simulink model "Q0107tsmc_egtsmc_egftsmc_final_sensitivity"  (R2024b)
settings: Solver=ode4  StartTime=0.0  StopTime=12  FixedStep=0.01  RelTol=1e-3  EnableMultiTasking=on
model workspace (MAT data in the model file):
  A1 = 0.0190784648009
  A2 = 0.089786568484
  B1 = 2.58582251419
  B2 = 0.593361860386
  Count = 20
  I1 = 0.276
  I2 = 0.0235
  I3 = 0.0235
  L1 = 0.5
  L2 = 0.4
  Lp1d = 0.49
  Lp2d = 0.39
  Lp3d = 0.39
  Tmax = 0
  Tmin = -1567
  alpha1 = 1.4711
  alpha2 = 1.4464
  b10 = 33.49
  b11 = 1.435
  b12 = 3.205e-06
  b13 = -161.2
  b14 = 3.294
  b15 = -1.575e-05
  d10 = -0.78
  d11 = -76.79
  d20 = -0.4716
  d21 = 0.47
  dq = [1.72653408644e-22 0.000273900412394 0.000547772970539 0.000821597382973 0.00109535342539 0.0013690210252 0.00164258022129 0.0019160110909 0.00218929391546 0.0024624089498 0.00273533666065 0.00300805756768 ... (1200 elements, 400x3)]
  f10 = 0.0038
  f11 = 141.13
  f20 = 0.0012
  f21 = 150.24
  fai1d = 0.03998
  fai2d = 0.01996
  fai3d = 0.01996
  fce10 = 164.4
  fec11 = 0.003852
  fec12 = -0.9149
  g = 9.8
  ii = -1
  jj = 1
  k10 = 13640
  k11 = 0.05356
  k12 = -37.89
  kk = -1
  ks1 = 394.1176
  ks2 = 379.0476
  ll = 0
  m1 = 3.612
  m2 = 1.762
  nn = 0.1
  out = Simulink.SimulationOutput
  out.Data.e1a1 = [0 0.001 0.002 0.003 0.004 0.005 0.006 0.007 0.008 0.009 0.01 0.011 ... (100002 elements, 50001x2)]
  out.Data.e2a1 = [0 0.001 0.002 0.003 0.004 0.005 0.006 0.007 0.008 0.009 0.01 0.011 ... (100002 elements, 50001x2)]
  out.Data.e3a1 = [0 0.001 0.002 0.003 0.004 0.005 0.006 0.007 0.008 0.009 0.01 0.011 ... (100002 elements, 50001x2)]
  out.Data.eA.time = []
  out.Data.eA.signals(1).values = [-0.004 -0.00400000010084 -0.00400000032797 -0.00400000067029 -0.0040000011369 -0.0040000017214 -0.00400000242883 -0.00400000325577 -0.00400000420507 -0.00400000527491 -0.00400000646695 -0.00400000778026 ... (50001 elements, 1x1x50001)]
  out.Data.eA.signals(1).dimensions = [1 1]
  out.Data.eA.signals(1).label = ''
  out.Data.eA.signals(1).title = ''
  out.Data.eA.signals(1).plotStyle = 0
  out.Data.eA.signals(2).values = [-0.003 -0.00300000621897 -0.0030000202079 -0.00300004127373 -0.00300006996011 -0.00300010586131 -0.00300014927337 -0.00300019997164 -0.00300025811767 -0.00300032358654 -0.00300039646582 -0.00300047668549 ... (50001 elements, 1x1x50001)]
  out.Data.eA.signals(2).dimensions = [1 1]
  out.Data.eA.signals(2).label = ''
  out.Data.eA.signals(2).title = ''
  out.Data.eA.signals(2).plotStyle = 0
  out.Data.eA.signals(3).values = [-0.003 -0.00299997512007 -0.00299991915681 -0.00299983488381 -0.00299972012759 -0.00299957651247 -0.00299940285536 -0.00299920005628 -0.00299896747016 -0.002998705598 -0.00299841409068 -0.00299809322965 ... (50001 elements, 1x1x50001)]
  out.Data.eA.signals(3).dimensions = [1 1]
  out.Data.eA.signals(3).label = ''
  out.Data.eA.signals(3).title = ''
  out.Data.eA.signals(3).plotStyle = 0
  out.Data.eA.blockName = 'HMPIDXXXGA1untitledqidongjirou33/Scope12'
  out.Data.tout = [0 0.001 0.002 0.003 0.004 0.005 0.006 0.007 0.008 0.009 0.01 0.011 ... (50001 elements, 50001x1)]
  out.Metadata = Simulink.SimulationMetadata
  out.Metadata.ModelInfo.ModelName = 'HMPIDXXXGA1untitledqidongjirou33'
  out.Metadata.ModelInfo.ModelVersion = '1.79'
  out.Metadata.ModelInfo.ModelFilePath = 'C:\Users\Administrator\Desktop\qidongjirou\5.22\HMPIDXXXGA1untitledqidongjirou33.slx'
  out.Metadata.ModelInfo.UserID = 'Administrator'
  out.Metadata.ModelInfo.MachineName = 'WIN-TQE2NG5IKIE'
  out.Metadata.ModelInfo.Platform = 'PCWIN64'
  out.Metadata.ModelInfo.ModelStructuralChecksum = [1369709381; 2978498901; 2960340512; 2746880361]
  out.Metadata.ModelInfo.SimulationMode = 'normal'
  out.Metadata.ModelInfo.StartTime = 0
  out.Metadata.ModelInfo.StopTime = 50
  out.Metadata.ModelInfo.SolverInfo.Type = 'Fixed-Step'
  out.Metadata.ModelInfo.SolverInfo.Solver = 'ode4'
  out.Metadata.ModelInfo.SolverInfo.FixedStepSize = 0.001
  out.Metadata.ModelInfo.SimulinkVersion.Name = 'Simulink'
  out.Metadata.ModelInfo.SimulinkVersion.Version = '10.6'
  out.Metadata.ModelInfo.SimulinkVersion.Release = '(R2022b)'
  out.Metadata.ModelInfo.SimulinkVersion.Date = '13-May-2022'
  out.Metadata.ModelInfo.LoggingInfo.LoggingToFile = 'off'
  out.Metadata.TimingInfo.WallClockTimestampStart = '2024-05-28 16:50:20'
  out.Metadata.TimingInfo.WallClockTimestampStop = '2024-05-28 16:50:25'
  out.Metadata.TimingInfo.InitializationElapsedWallTime = 0.7839932
  out.Metadata.TimingInfo.ExecutionElapsedWallTime = 4.4201347
  out.Metadata.TimingInfo.TerminationElapsedWallTime = 0.0157048
  out.Metadata.TimingInfo.TotalElapsedWallTime = 5.2198327
  out.Metadata.TimingInfo.ProfilerData = '探查器未启用'
  out.Metadata.ExecutionInfo.StopEvent = 'ReachedStopTime'
  out.Metadata.ExecutionInfo.StopEventSource = []
  out.Metadata.ExecutionInfo.StopEventDescription = '已达到 50 的停止时间'
  out.Metadata.ExecutionInfo.ErrorDiagnostic = []
  out.Metadata.ExecutionInfo.WarningDiagnostics.Diagnostic = MSLDiagnostic
  out.Metadata.ExecutionInfo.WarningDiagnostics.Diagnostic.identifier = 'Simulink:Engine:DefaultDimsMethodUsed'
  out.Metadata.ExecutionInfo.WarningDiagnostics.Diagnostic.message : char (value not decoded)
  out.Metadata.ExecutionInfo.WarningDiagnostics.Diagnostic.paths = {'HMPIDXXXGA1untitledqidongjirou33'}
  out.Metadata.ExecutionInfo.WarningDiagnostics.Diagnostic.arguments{1} = 'HMPIDXXXGA1untitledqidongjirou33'
  out.Metadata.ExecutionInfo.WarningDiagnostics.Diagnostic.arguments{2} : char (value not decoded)
  out.Metadata.ExecutionInfo.WarningDiagnostics.Diagnostic.stack = struct([])
  out.Metadata.ExecutionInfo.WarningDiagnostics.Diagnostic.priority = 2
  out.Metadata.ExecutionInfo.WarningDiagnostics.SimulationPhase = 'Initialization'
  out.Metadata.ExecutionInfo.WarningDiagnostics.SimulationTime = []
  out.Metadata.AppInfo = struct()
  p0 = 0
  q = [4.04864701555e-21 2.889959974e-21 2.73900412394e-06 8.21673382933e-06 1.64327076591e-05 2.7386241913e-05 4.1076452165e-05 5.75022543779e-05 7.66623652868e-05 9.85553044414e-05 0.000123179393939 0.000150532760546 ... (1200 elements, 400x3)]
  r = 0.05
  rhos0 = 76.79
  rhos1 = -1.54
  rhos2 = 0.4716
  rhos3 = 0.0969
  rhos4 = 78.21
  rhos5 = -1.6
  rhos6 = 0.3214
  rhos7 = 0.0821
  str = 'save 52216121_Testing20_data'
values from neighbouring files (symbols this model uses):
  A = 74.37    [AAAAA1195_data.mat]
  B = 0.18    [AAAAA1195_data.mat]
  d1 = 0.376115932997    [AAAAA1195_data.mat]
  d2 = 65.5377481102    [AAAAA1195_data.mat]
  gam1 = 1.36    [AAAAA1195_data.mat]
  gam2 = 1.23    [AAAAA1195_data.mat]
  ks = 23.13    [AAAAA1195_data.mat]
  kv = 12.52    [AAAAA1195_data.mat]
  q_expanded = [4.04864701555e-21 3.46930349477e-21 2.889959974e-21 1.36950206197e-06 2.73900412394e-06 5.47786897664e-06 8.21673382933e-06 1.23247207442e-05 1.64327076591e-05 2.1909474786e-05 2.7386241913e-05 3.4231347039e-05 ... (2400 elements, 800x3)]    [AAAAA1195_data.mat]
libraries: simulink x3
(part 1 of 2)
settings Model: Creator=Administrator  LastModifiedBy=ys
settings OptimizationCC: ReuseModelBlockBuffer=off
settings DebuggingCC: UnderSpecifiedDimensionMsg=warning
settings RTWCC: GPUComputeCapability=3.5

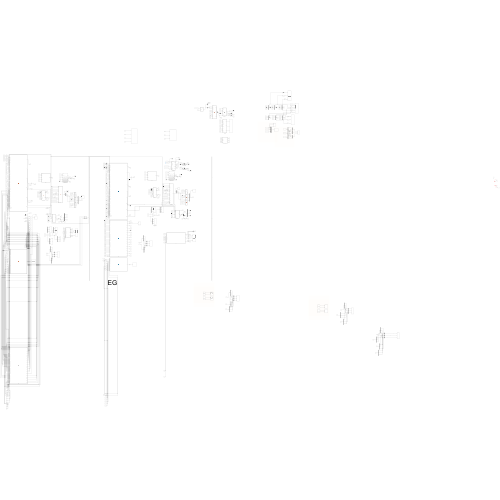
[thumbnail: Simulink's stored preview of the top-level diagram]
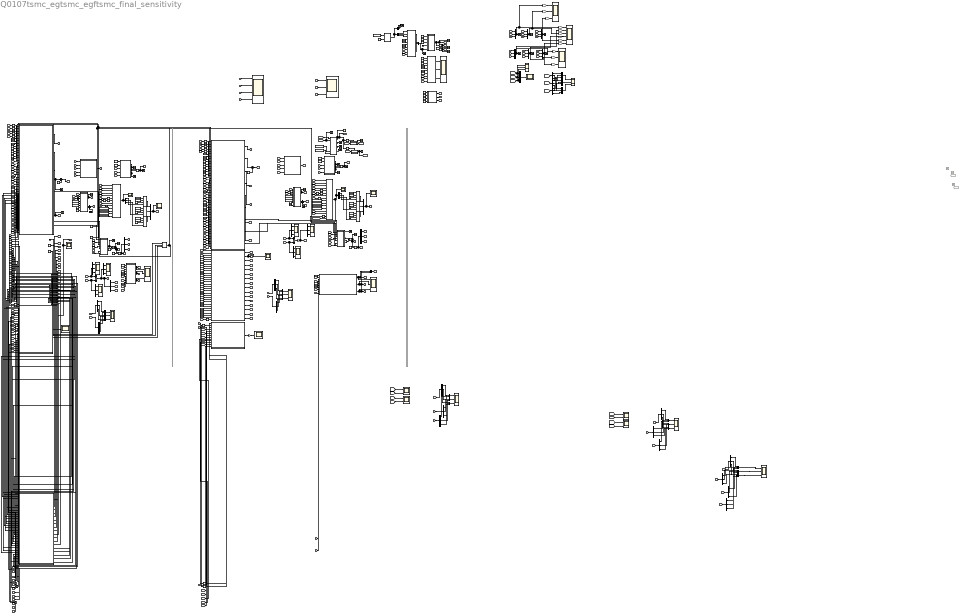
== system Q0107tsmc_egtsmc_egftsmc_final_sensitivity ==
  note: EG
  note: 预设长度
  note: 预设角度
  note: 误差显示
  Add1 : Sum  Inputs=+-
  Add3 : Sum  Inputs=+-
  Band-Limited White Noise1 : simulink/Sources/Band-Limited White Noise  Cov=[0.00025]  Ts=0.01  seed=[23341]
  Band-Limited White Noise3 : simulink/Sources/Band-Limited White Noise  Cov=[0.00025]  Ts=0.01  seed=[23341]
  Clock : Clock
  Constant{102,193,221,238,241,244} (6 alike) : Constant  Value=Tmin
  Constant{112,185,273,295} (4 alike) : Constant  Value=f21
  Constant113 : Constant  Value=Lp3d
  Constant{116,126,291,297} (4 alike) : Constant  Value=rhos4
  Constant119 : Constant  Value=Lp1d
  Constant120 : Constant  Value=Lp2d
  Constant{122,129,248,296} (4 alike) : Constant  Value=rhos6
  Constant127 : Constant  Value=f11
  Constant128 : Constant  Value=I1
  Constant{31,37,130,142,180,202,249,267..268,285} (10 alike) : Constant  Value=L2
  Constant{131..132,250,255} (4 alike) : Constant  Value=I2
  Constant{133,200,257,282} (4 alike) : Constant  Value=d20
  Constant134 : Constant  Value=rhos1
  Constant{135,201,259,283} (4 alike) : Constant  Value=d21
  Constant{136,186,260,274} (4 alike) : Constant  Value=m2
  Constant137 : Constant  Value=rhos3
  Constant{35,138..139,262..263} (5 alike) : Constant  Value=L1
  Constant{140,183,265,271} (4 alike) : Constant  Value=rhos5
  Constant{141,184,266,272} (4 alike) : Constant  Value=rhos7
  Constant15 : Constant  Value=Lp3d
  Constant16 : Constant  Value=Lp1d
  Constant181 : Constant  Value=f10
  Constant182 : Constant  Value=m1
  Constant{187,196,222,239,242,245} (6 alike) : Constant  Value=nn
  Constant{188,194,275,279} (4 alike) : Constant  Value=f20
  Constant189 : Constant  Value=p0
  Constant190 : Constant  Value=d10
  Constant{34,36,191,210,252,278,340} (7 alike) : Constant  Value=r
  Constant{99,192,220,237,240,243} (6 alike) : Constant  Value=Tmax
  Constant195 : Constant  Value=ks1
  Constant199 : Constant  Value=d11
  Constant{32..33,49,53,209,215,251,254,290,294,342..343} (12 alike) : Constant  Value=alpha2
  Constant{30,211,214,253,288,341} (6 alike) : Constant  Value=alpha1
  Constant212 : Constant  Value=rhos0
  Constant{52,213,287,293} (4 alike) : Constant  Value=ks2
  Constant223 : Constant  Value=kv
  Constant232 : Constant  Value=0.0095
  Constant233 : Constant  Value=A
  Constant234 : Constant  Value=ks
  Constant235 : Constant  Value=gam1
  Constant236 : Constant  Value=B
  Constant246 : Constant  Value=kv
  Constant247 : Constant  Value=A
  Constant256 : Constant  Value=ks
  Constant258 : Constant  Value=rhos1
  Constant261 : Constant  Value=rhos3
  Constant264 : Constant  Value=gam1
  Constant269 : Constant  Value=f10
  Constant27 : Constant  Value=Lp2d
  Constant270 : Constant  Value=m1
  Constant276 : Constant  Value=p0
  Constant277 : Constant  Value=d10
  Constant{28,80,284,306} (4 alike) : Constant
  Constant280 : Constant  Value=ks1
  Constant281 : Constant  Value=d11
  Constant286 : Constant  Value=rhos0
  Constant289 : Constant  Value=rhos2
  Constant292 : Constant  Value=g
  Constant298 : Constant  Value=gam2
  Constant{89,92,299,304} (4 alike) : Constant  Value=0
  Constant300 : Constant  Value=f11
  Constant301 : Constant  Value=I1
  Constant302 : Constant  Value=d1
  Constant303 : Constant  Value=d2
  Constant305 : Constant  Value=[0.500;0.400;0.400]
  Constant307 : Constant  Value=0.000000412
  Constant345 : Constant  Value=q_expanded
  Constant39 : Constant  Value=gam2
  Constant42 : Constant  Value=rhos2
  Constant50 : Constant  Value=g
  Constant94 : Constant  Value=d1
  Constant95 : Constant  Value=d2
  Constant96 : Constant  Value=B
  Constant97 : Constant  Value=[0.500;0.400;0.400]
  Counter Free-Running : simulink/Sources/Counter Free-Running  NumBits=16  tsamp=-1
  Demux{,1..7,9..13,15,20..21,24,26..30,39..46} (30 alike) : Demux  Outputs=3
  Demux19 : Demux  Commented=on  Outputs=3
  Demux8 : Demux  Commented=on  Outputs=3
  Derivative{5..8,12,15..16,27..30,39..55} (28 alike) : Derivative
  DisturbanceForceReference : Constant  Value=[407.077590693713;285.374396655646;71.2180167722357]
  DisturbanceFraction : Constant  Value=0
  DisturbanceTime : Clock
  Fp1输出1 : MATLAB Function  TreatAsAtomicUnit=on
  Fp1输出4 : MATLAB Function  TreatAsAtomicUnit=on
  Function-Call Subsystem2 : Subsystem  TreatAsAtomicUnit=on
  Function-Call Subsystem3 : Subsystem  TreatAsAtomicUnit=on
  Gain{5..16} (12 alike) : Gain  Gain=1000
  Gain2 : Gain  Gain=-1
  Gain3 : Gain  Gain=-1
  Goto122 : Goto  Commented=on  GotoTag=eiBB
  Goto125 : Goto  Commented=on  GotoTag=lastUfBB
  Integrator10 : Integrator
  Integrator{4,7,9,11} (4 alike) : Integrator  InitialConditionSource=external
  Integrator8 : Integrator
  Lx1 : MATLAB Function  TreatAsAtomicUnit=on
  Lx2 : MATLAB Function  TreatAsAtomicUnit=on
  Lx4 : MATLAB Function  TreatAsAtomicUnit=on
  MATLAB Function10 : MATLAB Function  TreatAsAtomicUnit=on
  MATLAB Function11 : MATLAB Function  TreatAsAtomicUnit=on
  MATLAB Function12 : MATLAB Function  TreatAsAtomicUnit=on
  MATLAB Function13 : MATLAB Function  TreatAsAtomicUnit=on
  MATLAB Function14 : MATLAB Function  TreatAsAtomicUnit=on
  MATLAB Function16 : MATLAB Function  TreatAsAtomicUnit=on
  MATLAB Function18 : MATLAB Function  TreatAsAtomicUnit=on
  MATLAB Function19 : MATLAB Function  TreatAsAtomicUnit=on
  MATLAB Function20 : MATLAB Function  TreatAsAtomicUnit=on
  MATLAB Function28 : MATLAB Function  TreatAsAtomicUnit=on
  MATLAB Function29 : MATLAB Function  TreatAsAtomicUnit=on
  MATLAB Function3 : MATLAB Function  TreatAsAtomicUnit=on
  MATLAB Function5 : MATLAB Function  TreatAsAtomicUnit=on
  MATLAB Function6 : MATLAB Function  TreatAsAtomicUnit=on
  MATLAB Function9 : MATLAB Function  TreatAsAtomicUnit=on
  Memory{1..2,7,10..11} (5 alike) : Memory
  Mux{,1..9,12..14,16,25..27,32..34} (20 alike) : Mux  Inputs=3
  Mux{10..11,15,17..19} (6 alike) : Mux  Inputs=2
  Mux35 : Mux
  Mux36 : Mux
  Mux37 : Mux
  PlantMassInertiaDelta : Constant  Value=0
  PlantStiffnessDelta : Constant  Value=0
  PrescribedExternalDisturbance : MATLAB Function  TreatAsAtomicUnit=on
  Product1 : Product  Multiplication=Matrix(*)
  Product4 : Product  Multiplication=Matrix(*)
  Scope{,1,3,7,12..13,15,39..41,51,53,58,69,76,80,82,103,107,111} (20 alike) : Scope  NumInputPorts=3
  Scope{37,50,101..102} (4 alike) : Scope  NumInputPorts=2
  Scope{5..6,8,23,29..30,34..35,38,42..49,52,54..56,61..63,65,67..68,75,77..79,81,83,85..86,90,104..106,108} (40 alike) : Scope
  Scope57 : Scope  NumInputPorts=6
  Scope87 : Scope  Commented=on
  Scope91 : Scope  Commented=on
  Scope93 : Scope  Commented=on
  Scope96 : Scope  NumInputPorts=4
  Step2 : Step  Before=0.00001  After=0  SampleTime=0
  Step3 : Step  Before=0.00001  After=0  SampleTime=0
  Sum{2..3,6,8} (4 alike) : Sum  Inputs=|++
  XBB1 : MATLAB Function  TreatAsAtomicUnit=on
  XBB3 : MATLAB Function  TreatAsAtomicUnit=on
  lambc1 : MATLAB Function  TreatAsAtomicUnit=on
  lambc4 : MATLAB Function  TreatAsAtomicUnit=on
  pso-RBF神经网络1 : Subsystem
  pso-RBF神经网络4 : Subsystem
  事件触发条件1 : MATLAB Function  TreatAsAtomicUnit=on
  滑模面2 : MATLAB Function  TreatAsAtomicUnit=on
  滑模面4 : MATLAB Function  TreatAsAtomicUnit=on
  计算Lpi2 : MATLAB Function  TreatAsAtomicUnit=on
  wires:
  Constant35/1 -> Lx1/2(L1)
  Constant37/1 -> Lx1/3(L2)
  Constant34/1 -> Lx1/1(r)
  Lx1/3(Lx3) -> [Lx3]
  Lx1/2(Lx2) -> [Lx2]
  Lx1/1(Lx1) -> [Lx1]
  Constant31/1 -> Lx1/4(L3)
  Constant15/1 -> MATLAB Function6/3(Lp3d)
  Clock/1 -> MATLAB Function5/4(t)
  Constant32/1 -> MATLAB Function6/5(alpha2)
  Constant36/1 -> MATLAB Function6/7(r)
  Derivative8/1 -> Scope6/1, [ddxd]
  [Lx1] -> MATLAB Function6/8(Lx1)
  Constant33/1 -> MATLAB Function6/6(alpha3)
  Constant27/1 -> MATLAB Function6/2(Lp2d)
  [Lx2] -> MATLAB Function6/9(Lx2)
  Derivative7/1 -> Scope8/1, [dxd], Derivative8/1
  MATLAB Function6/1(fai1dd) -> Scope7/1
  [Lx3] -> MATLAB Function6/10(Lx3)
  Constant30/1 -> MATLAB Function6/4(alpha1)
  Constant16/1 -> MATLAB Function6/1(Lp1d)
  Constant113/1 -> MATLAB Function5/3(Lp3d)
  MATLAB Function5/1(xd) -> Derivative7/1, Scope5/1, [xd]
  MATLAB Function6/3(fai3dd) -> Scope7/3
  Constant120/1 -> MATLAB Function5/2(Lp2d)
  Constant119/1 -> MATLAB Function5/1(Lp1d)
  MATLAB Function6/2(fai2dd) -> Scope7/2
  Demux21/2 -> Scope39/2
  Demux12/2 -> [Lp2B]
  [Lp3B] -> Derivative6/1
  lambc1/3(bp1) -> [bp1B]
  Constant140/1 -> lambc1/18(rhos5)
  [fai3B] -> MATLAB Function11/17(fai3)
  [Lp1B] -> lambc1/1(Lp1)
  lambc1/6(bp4) -> [bp4B]
  [Lp1B] -> MATLAB Function11/18(Lp1)
  lambc1/8(bp6) -> [bp6B]
  Constant195/1 -> MATLAB Function11/25(ks1)
  Constant137/1 -> lambc1/16(rhos3)
  Constant201/1 -> lambc1/31(d31)
  [Lp1B] -> Derivative16/1
  Constant133/1 -> lambc1/30(d30)
  [bp11B] -> MATLAB Function11/42(bp11)
  Constant185/1 -> lambc1/12(f31)
  Constant180/1 -> lambc1/5(L2)
  [lastUfB] -> Memory2/1
  Constant97/1 -> Integrator7/2
  Constant135/1 -> lambc1/29(d21)
  [bp12B] -> MATLAB Function11/43(bp12)
  lambc1/10(bp8) -> [bp8B]
  [Lp2B] -> lambc1/2(Lp2)
  Demux13/3 -> Scope41/3
  [fai1B] -> MATLAB Function11/15(fai1)
  [Lp3B] -> lambc1/3(Lp3)
  Constant112/1 -> lambc1/10(f21)
  Constant138/1 -> lambc1/4(L1)
  Constant202/1 -> lambc1/6(L3)
  Constant183/1 -> lambc1/22(rhos9)
  Constant184/1 -> lambc1/24(rhos11)
  Constant132/1 -> MATLAB Function11/7(I2)
  MATLAB Function11/1(Cf) -> [CfB]
  Constant50/1 -> MATLAB Function11/31(g)
  Constant139/1 -> MATLAB Function11/9(L1)
  lambc1/14(bp12) -> [bp12B]
  Constant200/1 -> lambc1/28(d20)
  Constant199/1 -> lambc1/27(d11)
  Constant212/1 -> lambc1/13(rhos0)
  Integrator7/1 -> [xB], Demux12/1
  Demux21/3 -> Scope39/3
  lambc1/5(bp3) -> [bp3B]
  [Lp2B] -> MATLAB Function11/19(Lp2)
  [bp3B] -> MATLAB Function11/34(bp3)
  Constant134/1 -> lambc1/14(rhos1)
  Constant214/1 -> MATLAB Function11/28(alpha1)
  Constant141/1 -> lambc1/20(rhos7)
  Add1/1 -> Gain2/1
  [bp6B] -> MATLAB Function11/37(bp6)
  [UfB] -> 计算Lpi2/2(Uf)
  lambc1/7(bp5) -> [bp5B]
  Demux20/3 -> Scope40/3
  Demux13/2 -> Scope41/2
  lambc1/1(Os) -> [OsB]
  Constant126/1 -> lambc1/21(rhos8)
  Constant130/1 -> MATLAB Function11/11(L3)
  Constant89/1 -> Integrator4/2
  [bp10B] -> MATLAB Function11/41(bp10)
  [bp5B] -> MATLAB Function11/36(bp5)
  lambc1/9(bp7) -> [bp7B]
  [xB] -> Add1/2, Demux21/1
  Demux20/2 -> Scope40/2
  Constant188/1 -> lambc1/9(f20)
  Constant181/1 -> lambc1/7(f10)
  Derivative15/1 -> MATLAB Function11/2(defai3)
  Constant53/1 -> MATLAB Function11/30(alpha3)
  [Lx3] -> MATLAB Function11/24(Lx3)
  Constant190/1 -> lambc1/26(d10)
  Constant42/1 -> lambc1/15(rhos2)
  lambc1/4(bp2) -> [bp2B]
  Derivative6/1 -> MATLAB Function11/5(deLp3)
  Constant129/1 -> lambc1/23(rhos10)
  Constant189/1 -> lambc1/25(p0)
  Constant116/1 -> lambc1/17(rhos4)
  Constant122/1 -> lambc1/19(rhos6)
  Constant127/1 -> lambc1/8(f11)
  Demux13/1 -> Scope41/1
  lambc1/11(bp9) -> [bp9B]
  Derivative16/1 -> MATLAB Function11/3(deLp1)
  [bp8B] -> MATLAB Function11/39(bp8)
  [bp7B] -> MATLAB Function11/38(bp7)
  [bp9B] -> MATLAB Function11/40(bp9)
  lambc1/13(bp11) -> [bp11B]
  Demux21/1 -> Scope39/1
  MATLAB Function11/6(Mf) -> [MfB]
  Constant194/1 -> lambc1/11(f30)
  Derivative5/1 -> MATLAB Function11/4(deLp2)
  Derivative12/1 -> MATLAB Function11/1(defai2)
  Constant136/1 -> MATLAB Function11/14(m3)
  Constant191/1 -> MATLAB Function11/21(r)
  [fai3B] -> Derivative15/1
  [bp4B] -> MATLAB Function11/35(bp4)
  [bp1B] -> MATLAB Function11/32(bp1)
  Constant182/1 -> MATLAB Function11/12(m1)
  [Lp3B] -> MATLAB Function11/20(Lp3)
  lambc1/12(bp10) -> [bp10B]
  Demux20/1 -> Scope40/1
  Constant52/1 -> MATLAB Function11/27(ks3)
  [Lx2] -> MATLAB Function11/23(Lx2)
  MATLAB Function11/2(Gf) -> Sum6/1
  [Lp2B] -> Derivative5/1
  [fai2B] -> MATLAB Function11/16(fai2)
  Demux12/1 -> [Lp1B]
  Constant128/1 -> MATLAB Function11/6(I1)
  Constant49/1 -> MATLAB Function11/29(alpha2)
  Constant142/1 -> MATLAB Function11/10(L2)
  [fai2B] -> Derivative12/1
  Constant213/1 -> MATLAB Function11/26(ks2)
  Constant131/1 -> MATLAB Function11/8(I3)
  [dxB] -> 计算Lpi2/4(dx)
  Demux12/3 -> [Lp3B]
  [bp2B] -> MATLAB Function11/33(bp2)
  [Lx1] -> MATLAB Function11/22(Lx1)
  [xd] -> Add1/1, Demux20/1
  Constant186/1 -> MATLAB Function11/13(m2)
  [OsB] -> 计算Lpi2/6(Os)
  Gain2/1 -> Demux13/1, [eB]
  [e1B] -> Mux/2
  [e1C] -> Mux/3
  [e1] -> Mux/1
  Mux/1 -> Gain6/1, Gain11/1, Scope34/1
  Mux4/1 -> Gain12/1, Gain8/1, Scope38/1
  [e2] -> Mux4/1
  [e2C] -> Mux4/3
  [e2B] -> Mux4/2
  [e3B] -> Mux5/2
  [e3C] -> Mux5/3
  [e3] -> Mux5/1
  Mux5/1 -> Gain13/1, Gain10/1, Scope47/1
  [PB] -> Scope53/2, Mux6/2
  [P] -> Scope53/1, Mux6/1
  [PC] -> Scope53/3, Mux6/3
  Mux6/1 -> Scope48/1
  Derivative27/1 -> MATLAB Function16/2(dLp2)
  lambc1/15(B1) -> [B1B]
  lambc1/16(B2) -> [B2B]
  [bp4B] -> MATLAB Function16/4(bp4)
  [bp6B] -> MATLAB Function16/6(bp6)
  [B1B] -> MATLAB Function16/8(B1)
  [PB] -> MATLAB Function16/10(P)
  MATLAB Function16/1(Fp) -> Gain3/1
  Gain3/1 -> Scope49/1
  MATLAB Function11/5(G3) -> [G3B]
  MATLAB Function11/4(G2) -> [G2B]
  MATLAB Function11/3(G1) -> [G1B]
  [G2B] -> MATLAB Function16/12(G2)
  [Lp1] -> Mux7/1
  [Lp1B] -> Mux7/2
  [Lp1C] -> Mux7/3
  Mux7/1 -> Gain16/1, Gain5/1, Scope54/1
  Mux8/1 -> Gain15/1, Gain7/1, Scope55/1
  [Lp2C] -> Mux8/3
  [Lp2B] -> Mux8/2
  [Lp2] -> Mux8/1
  [Lp3] -> Mux9/1
  [Lp3B] -> Mux9/2
  [Lp3C] -> Mux9/3
  Mux9/1 -> Gain14/1, Gain9/1, Scope56/1
  Gain5/1 -> Scope57/1
  Gain6/1 -> Scope57/2
  Gain7/1 -> Scope57/3
  Gain8/1 -> Scope57/4
  Gain9/1 -> Scope57/5
  Gain10/1 -> Scope57/6
  lambc1/2(U) -> [PB], Scope35/1
  Gain11/1 -> Scope13/1
  Gain13/1 -> Scope13/3
  Gain12/1 -> Scope13/2
  Gain14/1 -> Scope12/3
  Gain15/1 -> Scope12/2
  Gain16/1 -> Scope12/1
  [P] -> Demux1/1
  [PB] -> Demux5/1
  [PC] -> Demux6/1
  Demux1/1 -> Mux1/1
  Demux5/1 -> Mux1/2
  Demux6/1 -> Mux1/3
  Demux1/2 -> Mux2/1
  Demux5/2 -> Mux2/2
  Demux6/2 -> Mux2/3
  Demux1/3 -> Mux3/1
  Demux5/3 -> Mux3/2
  Demux6/3 -> Mux3/3
  Mux1/1 -> Scope15/1
  Mux2/1 -> Scope15/2
  Mux3/1 -> Scope15/3
  [dxd] -> XBB1/2(dxd)
  [xB] -> XBB1/5(xB)
  pso-RBF神经网络1/2(gujiw) -> Product1/1, Scope43/1
  [ddxd] -> XBB1/1(ddxd)
  Constant80/1 -> pso-RBF神经网络1/2(pop(i,2))
  [MfB] -> pso-RBF神经网络1/5(Mf)
  [sB] -> pso-RBF神经网络1/4(s)
  XBB1/1(xBB) -> [xBB]
  [xd] -> XBB1/3(xd)
  pso-RBF神经网络1/1(phix) -> Scope45/1, Product1/2
  [xBB] -> pso-RBF神经网络1/3(x)
  Product1/1 -> [fxB], Scope44/1
  Constant28/1 -> pso-RBF神经网络1/1(pop(i,1))
  [dxB] -> XBB1/4(dxB)
  [Lp3B] -> Lx4/10(Lp3)
  Constant210/1 -> Lx4/1(r)
  [Lx1] -> Lx4/2(Lx1)
  Constant209/1 -> Lx4/7(alpha3)
  [Lp1B] -> Lx4/8(Lp1)
  Lx4/3(fai3) -> Mux14/3, [fai3B], Scope69/3
  Lx4/1(fai1) -> Mux14/1, [fai1B], Scope69/1
  Lx4/2(fai2) -> Mux14/2, [fai2B], Scope69/2
  Constant215/1 -> Lx4/6(alpha2)
  Constant211/1 -> Lx4/5(alpha1)
  [Lx3] -> Lx4/4(Lx3)
  [fxB] -> Fp1输出1/16(fx)
  Constant220/1 -> MATLAB Function3/1(Tmax)
  Constant196/1 -> MATLAB Function9/3(nn)
  Derivative42/1 -> Fp1输出1/6(ddxd)
  Constant187/1 -> MATLAB Function10/3(nn)
  Derivative39/1 -> 滑模面2/2(de)
  Memory10/1 -> Fp1输出1/15(last_Uf)
  Derivative41/1 -> Fp1输出1/5(dx)
  [eB] -> Derivative39/1
  [GfB] -> Fp1输出1/3(Gf)
  Constant222/1 -> MATLAB Function3/3(nn)
  Constant235/1 -> 滑模面2/7(gam1)
  Derivative28/1 -> Derivative42/1
  Mux12/1 -> Scope23/1, [UfB]
  MATLAB Function3/1(TT) -> Mux12/3
  [eB] -> Fp1输出1/13(e)
  Constant99/1 -> MATLAB Function10/1(Tmax)
  MATLAB Function10/1(TT) -> Mux12/2
  [xB] -> Derivative41/1
  Step2/1 -> Sum2/2
  Constant192/1 -> MATLAB Function9/1(Tmax)
  Constant233/1 -> 滑模面2/4(A)
  Sum2/1 -> [rousB]
  Constant234/1 -> Fp1输出1/10(ks)
  滑模面2/2(rous) -> Sum2/1
  [triggerB] -> Fp1输出1/14(trigger)
  [xd] -> Derivative28/1
  [rousB] -> Fp1输出1/4(rous)
  [eB] -> 滑模面2/1(e)
  [sB] -> Fp1输出1/7(s)
  Constant221/1 -> MATLAB Function3/2(Tmin)
  滑模面2/1(s) -> [sB], Scope29/1
  Constant102/1 -> MATLAB Function10/2(Tmin)
  Demux2/2 -> MATLAB Function10/4(T)
  Integrator8/1 -> 滑模面2/3(ie)
  [MfB] -> Fp1输出1/1(Mf)
  MATLAB Function9/1(TT) -> Mux12/1
  [eB] -> Integrator8/1
  Constant94/1 -> Fp1输出1/11(d1)
  Constant193/1 -> MATLAB Function9/2(Tmin)
  Constant39/1 -> 滑模面2/8(gam2)
  [CfB] -> Fp1输出1/2(Cf)
  Constant96/1 -> 滑模面2/5(B)
  Demux2/3 -> MATLAB Function3/4(T)
  Demux2/1 -> MATLAB Function9/4(T)
  Constant92/1 -> 滑模面2/6(C)
  [sB] -> Derivative40/1
  Derivative40/1 -> Fp1输出1/8(ds)
  Constant223/1 -> Fp1输出1/9(kv)
  Constant95/1 -> Fp1输出1/12(d2)
  Integrator9/1 -> Scope105/1, [dx], Integrator11/1
  Constant304/1 -> Integrator9/2
  [Uf] -> MATLAB Function12/2(Uf)
  MATLAB Function12/1(ddx) -> Scope104/1, Integrator9/1
  Demux3/2 -> [Lp2]
  Demux3/1 -> [Lp1]
  Constant305/1 -> Integrator11/2
  [dx] -> MATLAB Function12/4(dx)
  Demux3/3 -> [Lp3]
  [Os] -> MATLAB Function12/6(Os)
  Integrator11/1 -> [x], Demux3/1
  Constant280/1 -> MATLAB Function14/25(ks1)
  [bp12] -> MATLAB Function14/43(bp12)
  Demux27/1 -> Scope80/1
  Lx2/3(fai3) -> [fai3], Scope76/3
  Constant301/1 -> MATLAB Function14/6(I1)
  Constant250/1 -> MATLAB Function14/8(I3)
  [bp8] -> MATLAB Function14/39(bp8)
  Demux27/3 -> Scope80/3
  [Uf] -> Memory11/1
  Constant263/1 -> MATLAB Function14/9(L1)
  [Lx3] -> MATLAB Function14/24(Lx3)
  [Lp3] -> MATLAB Function13/10(Lp3)
  Derivative55/1 -> MATLAB Function14/3(deLp1)
  [bp9] -> MATLAB Function13/22(bp9)
  [bp11] -> MATLAB Function13/24(bp11)
  Demux28/2 -> [e2]
  [fai2] -> Derivative52/1
  Demux28/1 -> [e1]
  [lambc3] -> MATLAB Function13/3(lambc3)
  Constant254/1 -> Lx2/6(alpha2)
  Constant287/1 -> MATLAB Function14/26(ks2)
  [lambc1] -> MATLAB Function13/1(lambc1)
  Constant288/1 -> MATLAB Function14/28(alpha1)
  Constant249/1 -> MATLAB Function14/11(L3)
  Constant260/1 -> MATLAB Function14/14(m3)
  [fai3] -> MATLAB Function14/17(fai3)
  [bp5] -> MATLAB Function13/18(bp5)
  [lambs3] -> MATLAB Function13/6(lambs3)
  [bp5] -> MATLAB Function14/36(bp5)
  [Lp1] -> MATLAB Function13/8(Lp1)
  [bp3] -> MATLAB Function14/34(bp3)
  [bp1] -> MATLAB Function14/32(bp1)
  [bp10] -> MATLAB Function14/41(bp10)
  [bp1] -> MATLAB Function13/14(bp1)
  [bp7] -> MATLAB Function14/38(bp7)
  [Lp2] -> MATLAB Function14/19(Lp2)
  [Lp2] -> Derivative46/1
  [fai1] -> MATLAB Function14/15(fai1)
  [xd] -> Add3/2, Demux27/1
  Demux7/3 -> Scope51/3
  Constant278/1 -> MATLAB Function14/21(r)
  Derivative47/1 -> MATLAB Function14/5(deLp3)
  [Lx1] -> MATLAB Function14/22(Lx1)
  [fai3] -> Derivative53/1
  MATLAB Function13/1(Fp) -> Scope42/1
  [bp3] -> MATLAB Function13/16(bp3)
  Derivative44/1 -> MATLAB Function13/11(dLp1)
  Derivative51/1 -> MATLAB Function13/13(dLp3)
  [Lx2] -> MATLAB Function14/23(Lx2)
  Constant274/1 -> MATLAB Function14/13(m2)
  Derivative52/1 -> MATLAB Function14/1(defai2)
  [bp4] -> MATLAB Function14/35(bp4)
  [Lp1] -> MATLAB Function14/18(Lp1)
  Demux28/3 -> [e3]
  [bp7] -> MATLAB Function13/20(bp7)
  Add3/1 -> Demux7/1, [e], Demux28/1
  Constant255/1 -> MATLAB Function14/7(I2)
  [Lp3] -> MATLAB Function14/20(Lp3)
  Constant292/1 -> MATLAB Function14/31(g)
  [Lp3] -> Derivative47/1
  [fai2] -> MATLAB Function14/16(fai2)
  Constant294/1 -> MATLAB Function14/30(alpha3)
  [bp2] -> MATLAB Function14/33(bp2)
  Constant270/1 -> MATLAB Function14/12(m1)
  Constant293/1 -> MATLAB Function14/27(ks3)
  [bp11] -> MATLAB Function14/42(bp11)
  Constant267/1 -> MATLAB Function14/10(L2)
  [bp9] -> MATLAB Function14/40(bp9)
  MATLAB Function14/3(Mf) -> [Mf], Scope78/1
  MATLAB Function14/1(Cf) -> [Cf]
  [Lp1] -> Derivative55/1
  Demux7/1 -> Scope51/1
  Lx2/1(fai1) -> [fai1], Scope76/1
  Constant252/1 -> Lx2/1(r)
  Demux24/2 -> Scope82/2
  [x] -> Add3/1, Demux24/1
  Constant253/1 -> Lx2/5(alpha1)
  Demux7/2 -> Scope51/2
  [Lp2] -> Lx2/9(Lp2)
  Lx2/2(fai2) -> [fai2], Scope76/2
  Demux24/3 -> Scope82/3
  [Lx1] -> Lx2/2(Lx1)
  [Lx3] -> Lx2/4(Lx3)
  Demux27/2 -> Scope80/2
  Derivative53/1 -> MATLAB Function14/2(defai3)
  Demux24/1 -> Scope82/1
  [bp6] -> MATLAB Function14/37(bp6)
  Derivative46/1 -> MATLAB Function14/4(deLp2)
  Constant290/1 -> MATLAB Function14/29(alpha2)
  Mux13/1 -> [Uf], Scope62/1
  [e] -> 滑模面4/1(e)
  [s] -> Fp1输出4/8(s)
  Constant243/1 -> MATLAB Function18/1(Tmax)
  Derivative43/1 -> Derivative54/1
  Constant306/1 -> pso-RBF神经网络4/2(pop(i,2))
  Constant238/1 -> MATLAB Function20/2(Tmin)
  XBB3/1(xBB) -> [xAA1]
  MATLAB Function20/1(TT) -> Mux13/2
  Demux4/3 -> MATLAB Function18/4(T)
  Constant237/1 -> MATLAB Function20/1(Tmax)
  MATLAB Function19/1(TT) -> Mux13/1
  Integrator10/1 -> 滑模面4/3(ie)
  [Cf] -> Fp1输出4/3(Cf)
  [rous1] -> Fp1输出4/5(rous)
  Constant298/1 -> 滑模面4/8(gam2)
  Constant284/1 -> pso-RBF神经网络4/1(pop(i,1))
  [dx] -> XBB3/4(dxB)
  Demux4/1 -> MATLAB Function19/4(T)
  [s] -> pso-RBF神经网络4/4(s)
  Constant240/1 -> MATLAB Function19/1(Tmax)
  MATLAB Function18/1(TT) -> Mux13/3
  Constant244/1 -> MATLAB Function18/2(Tmin)
  Constant239/1 -> MATLAB Function20/3(nn)
  Demux4/2 -> MATLAB Function20/4(T)
  [Mf] -> pso-RBF神经网络4/5(Mf)
  Constant245/1 -> MATLAB Function18/3(nn)
  [xAA1] -> pso-RBF神经网络4/3(x)
  pso-RBF神经网络4/2(gujiw) -> Scope83/1, Product4/1
  pso-RBF神经网络4/1(phix) -> Product4/2, Scope52/1
  Product4/1 -> Scope46/1, [phifx]
  Fp1输出4/1(Uf) -> Scope77/1, Demux4/1
  [xd] -> XBB3/3(xd)
  [s] -> Derivative49/1
  Derivative49/1 -> Fp1输出4/9(ds)
  滑模面4/2(rous) -> Sum3/1
  [e] -> Integrator10/1
  Constant302/1 -> Fp1输出4/12(d1)
  滑模面4/1(s) -> Scope75/1, [s]
  Constant299/1 -> 滑模面4/6(C)
  [Mf] -> Fp1输出4/2(Mf)
  [x] -> Derivative50/1
  Constant241/1 -> MATLAB Function19/2(Tmin)
  Constant242/1 -> MATLAB Function19/3(nn)
  [dxd] -> XBB3/2(dxd)
  Sum3/1 -> [rous1]
  Constant303/1 -> Fp1输出4/13(d2)
  Constant236/1 -> 滑模面4/5(B)
  Derivative54/1 -> Fp1输出4/7(ddxd)
  Step3/1 -> Sum3/2
  [e] -> Derivative48/1
  Derivative48/1 -> 滑模面4/2(de)
  Derivative50/1 -> Fp1输出4/6(dx)
  Constant247/1 -> 滑模面4/4(A)
  Constant256/1 -> Fp1输出4/11(ks)
  [phifx] -> Fp1输出4/1(fx)
  [xd] -> Derivative43/1
  Constant264/1 -> 滑模面4/7(gam1)
  Constant246/1 -> Fp1输出4/10(kv)
  [x] -> XBB3/5(xB)
  [ddxd] -> XBB3/1(ddxd)
  [Gf] -> Fp1输出4/4(Gf)
  [mutA] -> Scope96/3
  [eA] -> Scope96/2
  [e] -> Scope96/1
  Fp1输出1/1(Uf) -> Memory10/1, Scope30/1, Demux2/1
  [P] -> Scope107/1
  [PA] -> Scope107/2
  [PC] -> Scope107/3
  [eC] -> Scope96/4
  [eiB] -> 事件触发条件1/1(sample_zeta_e)
  Function-Call Subsystem2/1(Out1) -> Scope68/1, [eiB]
  Memory7/1 -> Function-Call Subsystem2/Trigger
  [eB] -> Scope85/1, 事件触发条件1/2(e)
  事件触发条件1/2(ek) -> Scope86/1
  [eB] -> Function-Call Subsystem2/1(In1)
  事件触发条件1/3(norm_ek) -> Scope65/1
  Function-Call Subsystem3/1(Out1) -> [lastUfB], Scope61/1
  事件触发条件1/1(trigger) -> Memory1/1, Memory7/1, [triggerB], Scope63/1
  Memory1/1 -> Function-Call Subsystem3/Trigger
  [UfB] -> Function-Call Subsystem3/1(In1)
  事件触发条件1/4(threshold) -> Scope67/1
  Memory2/1 -> lambc1/32(Uf)
  Mux14/1 -> [faiB]
  [Lx3] -> MATLAB Function29/10(Lx3)
  [Lx2] -> MATLAB Function29/9(Lx2)
  [Lx1] -> MATLAB Function29/8(Lx1)
  Constant340/1 -> MATLAB Function29/7(r)
  Constant343/1 -> MATLAB Function29/6(alpha3)
  Constant342/1 -> MATLAB Function29/5(alpha2)
  Constant341/1 -> MATLAB Function29/4(alpha1)
  Demux/1 -> MATLAB Function29/1(phi1dd)
  Demux/2 -> MATLAB Function29/2(phi2dd)
  Demux/3 -> MATLAB Function29/3(phi3dd)
  MATLAB Function29/1(Lp1d) -> Mux16/1
  MATLAB Function29/2(Lp2d) -> Mux16/2
  MATLAB Function29/3(Lp3d) -> Mux16/3
  Mux16/1 -> Scope90/1, MATLAB Function5/5(yushe)
  MATLAB Function28/1(out) -> Demux42/1, Demux/1
  Constant345/1 -> MATLAB Function28/1(u)
  Counter Free-Running/1 -> MATLAB Function28/2(timeStepIdx)
  Demux10/2 -> Mux15/1
  Demux10/3 -> Mux17/1
  [xB] -> Demux15/1
  Demux15/2 -> Mux15/2
  [xd] -> Demux10/1
  Demux15/1 -> Mux11/2
  Demux10/1 -> Mux11/1
  Demux15/3 -> Mux17/2
  Mux11/1 -> Scope3/1
  Mux17/1 -> Scope3/3
  Mux15/1 -> Scope3/2
  Demux9/1 -> Mux10/1
  Mux18/1 -> Scope1/2
  Mux19/1 -> Scope1/3
  Demux11/3 -> Mux19/2
  Mux10/1 -> Scope1/1
  [xd] -> Demux9/1
  Demux9/3 -> Mux19/1
  Demux9/2 -> Mux18/1
  Demux11/2 -> Mux18/2
  Demux11/1 -> Mux10/2
  [x] -> Demux11/1
  [triggerB] -> Scope37/2
  [triggerCC] -> Scope37/1
  [PCC] -> Scope50/1
  [PB] -> Scope50/2
  Demux26/2 -> Mux26/1
  Demux26/3 -> Mux27/1
  [xCC] -> Demux29/1
  Demux29/2 -> Mux26/2
  [xd] -> Demux26/1
  Demux29/1 -> Mux25/2
  Demux26/1 -> Mux25/1
  Demux29/3 -> Mux27/2
  Mux25/1 -> Scope58/1
  Mux27/1 -> Scope58/3
  Mux26/1 -> Scope58/2
  [xB] -> Demux30/1
  Demux30/1 -> Mux25/3
  Demux30/2 -> Mux26/3
  Demux30/3 -> Mux27/3
  ? -> Scope93/1, Goto122/1
  ? -> Goto125/1, Scope87/1
  Mux33/1 -> Scope103/2
  Demux40/2 -> Mux33/2
  Mux34/1 -> Scope103/3
  Demux41/1 -> Mux32/3
  [xd] -> Demux39/1
  [PB] -> Scope102/2
  [triggerBB] -> Scope101/1
  Demux39/3 -> Mux34/1
  Demux41/3 -> Mux34/3
  [xBB1] -> Demux40/1
  Demux39/2 -> Mux33/1
  [xB] -> Demux41/1
  Demux39/1 -> Mux32/1
  [PBB] -> Scope102/1
  Demux40/1 -> Mux32/2
  Demux41/2 -> Mux33/3
  [triggerB] -> Scope101/2
  Demux40/3 -> Mux34/2
  Mux32/1 -> Scope103/1
  Integrator4/1 -> Scope108/1, [dxB], Integrator7/1
  计算Lpi2/1(ddx) -> Scope106/1, Integrator4/1
  Demux42/1 -> Scope/1
  Demux42/2 -> Scope/2
  Demux42/3 -> Scope/3
  Sum6/1 -> [GfB]
  Band-Limited White Noise1/1 -> Sum6/2
  Sum8/1 -> [Gf]
  MATLAB Function14/2(Gf) -> Sum8/1, Scope81/1
  Band-Limited White Noise3/1 -> Sum8/2
  Mux35/1 -> Scope111/1
  Demux44/3 -> Mux37/2
  Demux45/2 -> Mux36/3
  Demux44/1 -> Mux35/2
  Demux43/1 -> Mux35/1
  [xB] -> Demux45/1
  Demux43/2 -> Mux36/1
  [xBB1] -> Demux44/1
  Demux45/3 -> Mux37/3
  Demux43/3 -> Mux37/1
  [xd] -> Demux43/1
  Demux45/1 -> Mux35/3
  Mux37/1 -> Scope111/3
  Demux44/2 -> Mux36/2
  Mux36/1 -> Scope111/2
  [x] -> Demux46/1
  Demux46/1 -> Mux35/4
  Demux46/2 -> Mux36/4
  Demux46/3 -> Mux37/4
  Constant232/1 -> 事件触发条件1/7(sigma0)
  Constant307/1 -> 事件触发条件1/8(delta0)
  MATLAB Function11/9(MfPlant) -> 计算Lpi2/1(Mf)
  MATLAB Function11/7(CfPlant) -> 计算Lpi2/3(Cf)
  MATLAB Function11/8(GfPlant) -> 计算Lpi2/5(Gf)
  MATLAB Function14/6(MfPlant) -> MATLAB Function12/1(Mf)
  MATLAB Function14/4(CfPlant) -> MATLAB Function12/3(Cf)
  MATLAB Function14/5(GfPlant) -> MATLAB Function12/5(Gf)
  PlantStiffnessDelta/1 -> MATLAB Function14/45(deltaStiffness), MATLAB Function11/45(deltaStiffness)
  PlantMassInertiaDelta/1 -> MATLAB Function14/44(deltaMassInertia), MATLAB Function11/44(deltaMassInertia)
  [Lx2] -> Lx2/3(Lx2)
  [Lp3] -> Lx2/10(Lp3)
  [Lp1] -> Lx2/8(Lp1)
  Constant251/1 -> Lx2/7(alpha3)
  PrescribedExternalDisturbance/1(dExt) -> MATLAB Function12/7(dExt), 计算Lpi2/7(dExt)
  DisturbanceFraction/1 -> PrescribedExternalDisturbance/3(lambda)
  DisturbanceForceReference/1 -> PrescribedExternalDisturbance/2(U_nom)
  DisturbanceTime/1 -> PrescribedExternalDisturbance/1(t)
  lambc4/20(lambs3) -> [lambs3]
  Constant265/1 -> lambc4/18(rhos5)
  Constant281/1 -> lambc4/27(d11)
  lambc4/3(bp1) -> [bp1]
  [Lp3] -> lambc4/3(Lp3)
  Constant258/1 -> lambc4/14(rhos1)
  lambc4/10(bp8) -> [bp8]
  lambc4/14(bp12) -> [bp12]
  Constant300/1 -> lambc4/8(f11)
  lambc4/5(bp3) -> [bp3]
  lambc4/1(Os) -> [Os]
  lambc4/7(bp5) -> [bp5]
  lambc4/12(bp10) -> [bp10]
  lambc4/8(bp6) -> [bp6]
  Constant279/1 -> lambc4/11(f30)
  Constant261/1 -> lambc4/16(rhos3)
  lambc4/9(bp7) -> [bp7]
  [Lp3] -> Derivative51/1
  [bp12] -> MATLAB Function13/25(bp12)
  [Lp2] -> lambc4/2(Lp2)
  lambc4/19(lambs2) -> [lambs2]
  lambc4/16(lambc2) -> [lambc2]
  [Lp1] -> lambc4/1(Lp1)
  lambc4/15(lambc1) -> [lambc1]
  lambc4/18(lambs1) -> [lambs1]
  Constant262/1 -> lambc4/4(L1)
  Constant269/1 -> lambc4/7(f10)
  Constant259/1 -> lambc4/29(d21)
  Constant291/1 -> lambc4/17(rhos4)
  Constant297/1 -> lambc4/21(rhos8)
  [lambc2] -> MATLAB Function13/2(lambc2)
  Constant268/1 -> lambc4/5(L2)
  Constant289/1 -> lambc4/15(rhos2)
  lambc4/6(bp4) -> [bp4]
  Constant282/1 -> lambc4/28(d20)
  [lambs2] -> MATLAB Function13/5(lambs2)
  Constant285/1 -> lambc4/6(L3)
  lambc4/4(bp2) -> [bp2]
  Constant276/1 -> lambc4/25(p0)
  Constant266/1 -> lambc4/20(rhos7)
  Constant273/1 -> lambc4/12(f31)
  [lambs1] -> MATLAB Function13/4(lambs1)
  [bp4] -> MATLAB Function13/17(bp4)
  Constant257/1 -> lambc4/30(d30)
  Constant275/1 -> lambc4/9(f20)
  lambc4/17(lambc3) -> [lambc3]
  Constant248/1 -> lambc4/23(rhos10)
  Constant271/1 -> lambc4/22(rhos9)
  [Lp1] -> Derivative44/1
  Memory11/1 -> lambc4/32(Uf)
  [P] -> MATLAB Function13/7(p)
  Constant295/1 -> lambc4/10(f21)
  [bp2] -> MATLAB Function13/15(bp2)
  [bp6] -> MATLAB Function13/19(bp6)
  Derivative45/1 -> MATLAB Function13/12(dLp2)
  lambc4/13(bp11) -> [bp11]
  Constant277/1 -> lambc4/26(d10)
  lambc4/2(U) -> Scope79/1, [P]
  [Lp2] -> MATLAB Function13/9(Lp2)
  Constant272/1 -> lambc4/24(rhos11)
  lambc4/11(bp9) -> [bp9]
  [bp10] -> MATLAB Function13/23(bp10)
  [bp8] -> MATLAB Function13/21(bp8)
  Constant296/1 -> lambc4/19(rhos6)
  Constant283/1 -> lambc4/31(d31)
  [Lp2] -> Derivative45/1
  Constant286/1 -> lambc4/13(rhos0)
  [Lp2B] -> Lx4/9(Lp2)
  [Lx2] -> Lx4/3(Lx2)
  [G3B] -> MATLAB Function16/13(G3)
  [G1B] -> MATLAB Function16/11(G1)
  [B2B] -> MATLAB Function16/9(B2)
  [GfB] -> MATLAB Function16/7(Gf)
  [bp5B] -> MATLAB Function16/5(bp5)
  [Lp1B] -> Derivative30/1
  Derivative30/1 -> MATLAB Function16/1(dLp1)
  [Lp3B] -> Derivative29/1
  [Lp2B] -> Derivative27/1
  Derivative29/1 -> MATLAB Function16/3(dLp3)
